simulink model "ISAModel_TestModel"  (R2014a)
settings: Solver=ode45  StartTime=0.0  StopTime=300  RelTol=1e-3
libraries: rocket_isa_model_library x2, aerolibatmos2 x1, simulink x1
settings Model: Creator=scorpii  LastModifiedBy=scorpii

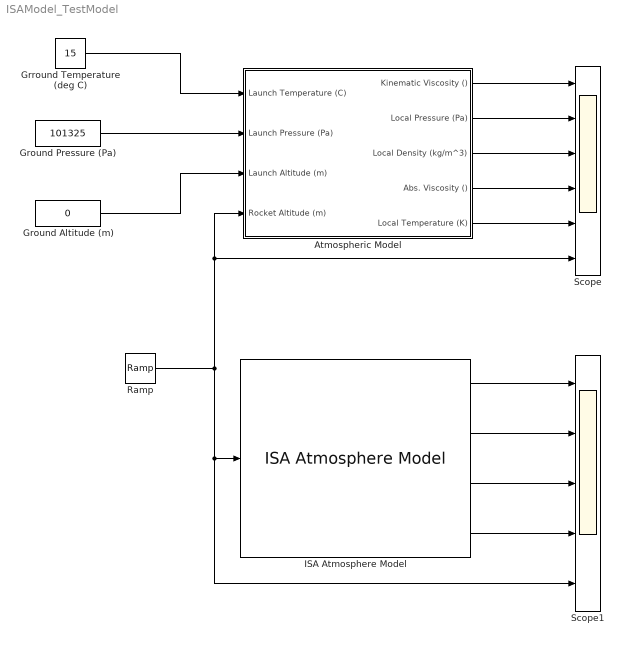
== system ISAModel_TestModel ==
  Atmospheric Model : Subsystem
  Ground Altitude (m) : Constant  Value=0
  Ground Pressure (Pa) : Constant  Value=101325
  Grround Temperature (deg C) : Constant  Value=15
  ISA Atmosphere Model : aerolibatmos2/ISA Atmosphere Model  custom=on  g=9.80665  gamma=1.4  R=287.0531  L=0.0065  h_trop=11000  h_strat=20000  rho0=1.225  P0=101325  T0=288.15  h0=0
  Ramp : simulink/Sources/Ramp  slope=1  start=0  X0=0
  Scope : Scope  NumInputPorts=6
      settings: YMin=-1.59652e-08~101325~23.5333~-3.75715e-07~15~-1  YMax=-1.59652e-08~101325~23.5333~-3.75715e-07~15~1
  Scope1 : Scope  NumInputPorts=5
      settings: YMin=-5~-5~-5~-5~-5  YMax=5~5~5~5~5
  wires:
  Ramp/1 -> Atmospheric Model/4(Rocket Altitude (m)), Scope/6, Scope1/5, ISA Atmosphere Model/1
  Grround Temperature (deg C)/1 -> Atmospheric Model/1(Launch Temperature (C))
  Ground Pressure (Pa)/1 -> Atmospheric Model/2(Launch Pressure (Pa))
  Atmospheric Model/1(Kinematic Viscosity ()) -> Scope/1
  Atmospheric Model/3(Local Density (kg/m^3)) -> Scope/3
  Atmospheric Model/2(Local Pressure (Pa)) -> Scope/2
  Atmospheric Model/5(Local Temperature (K)) -> Scope/5
  Atmospheric Model/4(Abs. Viscosity ()) -> Scope/4
  ISA Atmosphere Model/2 -> Scope1/2
  ISA Atmosphere Model/3 -> Scope1/3
  ISA Atmosphere Model/1 -> Scope1/1
  ISA Atmosphere Model/4 -> Scope1/4
  Ground Altitude (m)/1 -> Atmospheric Model/3(Launch Altitude (m))

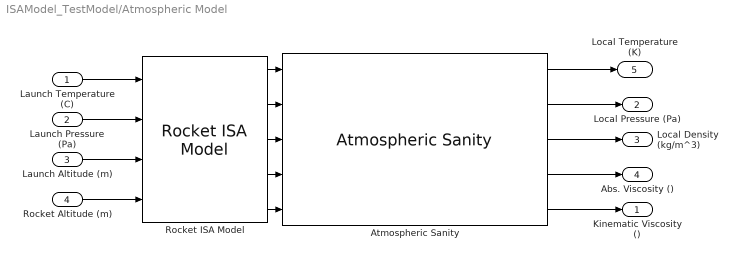
== system ISAModel_TestModel/Atmospheric Model ==
  Launch Temperature (C) : Inport
  Launch Pressure (Pa) : Inport  Port=2
  Launch Altitude (m) : Inport  Port=3
  Rocket Altitude (m) : Inport  Port=4
  Atmospheric Sanity : rocket_isa_model_library/Atmospheric Sanity
  Rocket ISA Model : rocket_isa_model_library/Rocket ISA Model
  Kinematic Viscosity () : Outport
  Local Pressure (Pa) : Outport  Port=2
  Local Density (kg/m^3) : Outport  Port=3
  Abs. Viscosity () : Outport  Port=4
  Local Temperature (K) : Outport  Port=5
  wires:
  Rocket ISA Model/5 -> Atmospheric Sanity/5
  Rocket ISA Model/2 -> Atmospheric Sanity/2
  Rocket ISA Model/3 -> Atmospheric Sanity/3
  Atmospheric Sanity/2 -> Local Pressure (Pa)/1
  Rocket ISA Model/4 -> Atmospheric Sanity/4
  Atmospheric Sanity/5 -> Kinematic Viscosity ()/1
  Atmospheric Sanity/1 -> Local Temperature (K)/1
  Atmospheric Sanity/3 -> Local Density (kg/m^3)/1
  Rocket ISA Model/1 -> Atmospheric Sanity/1
  Launch Temperature (C)/1 -> Rocket ISA Model/1
  Atmospheric Sanity/4 -> Abs. Viscosity ()/1
  Launch Pressure (Pa)/1 -> Rocket ISA Model/2
  Launch Altitude (m)/1 -> Rocket ISA Model/3
  Rocket Altitude (m)/1 -> Rocket ISA Model/4
